simulink model "atrias_nmm_hardware"  (R2014b)
settings: Solver=ode4  StartTime=0.0  StopTime=inf  FixedStep=sample_time  RelTol=1e-3
undefined symbols (not defined in the file): A_lpf_dtau, B1_lpf_dtau, B2_lpf_dtau, boom_mount_angle, boom_pelvis_offset_angle, c, c_jointstop, contactThr, control_start_time, D12_T, d_y_boom_com_offset, d_y_boom_hip_offset, eref, fcut_contact, FmaxBFSH, FmaxGLU, FmaxHAM, FmaxHFL, FmaxRF, FmaxVAS, g, h_boom, HIP_MTR_MAX_CONT_TORQUE, initial_com_height, initial_dx, K, k_sea, kd_lateral, kd_phi12, kd_phi23, kp_lateral, kp_phi12, kp_phi23, l_boom_projected, L_distribution_switch, L_force_ctrl_switch, L_hip_trq_desired, L_knee_trq_desired, L_sea_input_switch, l_seg, L_stim_gain, L_stim_switch, l_yaw_center_to_pelvis, lambdaHip, lambdaKnee, lateral_offset, lateral_target_angle_left, lateral_target_angle_right, lateral_transition_force, loptBFSH, loptGLU, loptHAM, loptHFL, loptRF, loptVAS, Lphi12_des, Lphi23_des, lslackBFSH, lslackGLU, lslackHAM ... (+69)
libraries: simulink_extras x15, simulink x5, slrtlib x3
(part 9 of 9)

== matlab function atrias_nmm_hardware/Control/Behavior Control/Lateral Control ==
  data: tau_r output size=1; qLateralR input; dqLateralR input; qLateralL input; dqLateralL input; F_leg_R input; F_leg_L input; L_leg_R input; L_leg_L input; lateral_transition_force parameter; lateral_target_angle_right parameter; lateral_target_angle_left parameter; boom_mount_angle parameter; boom_pelvis_offset_angle parameter; l_yaw_center_to_pelvis parameter; m_leg_motor parameter; g parameter; lateral_offset parameter; tau_l output size=1; kp_lateral parameter; kd_lateral parameter; minimum_lateral_angle parameter; maximum_lateral_angle parameter; HIP_MTR_MAX_CONT_TORQUE parameter
function [tau_r, tau_l] = LateralBoomControl(qLateralR, dqLateralR, qLateralL, dqLateralL, F_leg_R, F_leg_L, L_leg_R, L_leg_L, lateral_transition_force, lateral_target_angle_right, lateral_target_angle_left, boom_mount_angle, boom_pelvis_offset_angle, l_yaw_center_to_pelvis, m_leg_motor, g, lateral_offset, kp_lateral, kd_lateral, minimum_lateral_angle, maximum_lateral_angle, HIP_MTR_MAX_CONT_TORQUE)

    gravity_compensation = m_leg_motor*g*lateral_offset;
    if (F_leg_R < lateral_transition_force && F_leg_L < lateral_transition_force), gravity_compensation = 0; end % freefall
    
    % Right Leg
    desired = saturate([lateral_target_angle_right, 0],minimum_lateral_angle,maximum_lateral_angle);
    measured = [qLateralR, dqLateralR];
    tau_r = [kp_lateral, kd_lateral] * (desired-measured)' + gravity_compensation;
    tau_r = max(min(HIP_MTR_MAX_CONT_TORQUE, tau_r),-HIP_MTR_MAX_CONT_TORQUE);
    
    if (F_leg_R >= lateral_transition_force)
        angle = qLateralR - boom_pelvis_offset_angle + boom_mount_angle;
        J =   (L_leg_R - l_yaw_center_to_pelvis*sin(angle)) ./ (L_leg_R.*l_yaw_center_to_pelvis.*cos(angle) - l_yaw_center_to_pelvis*lateral_offset*sin(angle));    
        tau_r = -F_leg_R*(J - lateral_offset) + gravity_compensation;
    end
    
    % Left Leg
    desired = saturate([lateral_target_angle_left, 0],minimum_lateral_angle,maximum_lateral_angle);
    measured = [qLateralL, dqLateralL];
    tau_l = [kp_lateral, kd_lateral] * (desired-measured)' + gravity_compensation;
    tau_l = max(min(HIP_MTR_MAX_CONT_TORQUE, tau_l),-HIP_MTR_MAX_CONT_TORQUE);
    
    if (F_leg_L >= lateral_transition_force)
        angle = qLateralL + boom_pelvis_offset_angle - boom_mount_angle;
        J =  -(L_leg_L + l_yaw_center_to_pelvis*sin(angle)) ./ (L_leg_L.*l_yaw_center_to_pelvis.*cos(angle) - l_yaw_center_to_pelvis*lateral_offset*sin(angle));  
        tau_l = F_leg_L*(J - lateral_offset) + gravity_compensation;  
    end
    
    % Stance
%     if ~escape
%         if ~placement && right_or_left
%             angle = qLateralR - boom_pelvis_offset_angle + boom_mount_angle;
%             J =   (l_leg - l_yaw_center_to_pelvis*sin(angle)) ./ (l_leg.*l_yaw_center_to_pelvis.*cos(angle) - l_yaw_center_to_pelvis*lateral_offset*sin(angle));    
%             tau_r = -F_leg*(J - lateral_offset) + gravity_compensation; % + lateral_offset ???  -F*(J+r) + g       F*(J-r) + g
%         elseif ~placement && ~right_or_left
%             angle = qLateralL + boom_pelvis_offset_angle - boom_mount_angle;
%             J =  -(l_leg + l_yaw_center_to_pelvis*sin(angle)) ./ (l_leg.*l_yaw_center_to_pelvis.*cos(angle) - l_yaw_center_to_pelvis*lateral_offset*sin(angle));  
%             tau_l = F_leg*(J - lateral_offset) + gravity_compensation;
%         end
%     end
end

function [desired_saturated] = saturate(desired, minimum_lateral_angle, maximum_lateral_angle)
    desired_saturated = desired;
    if desired(1) < minimum_lateral_angle
        desired_saturated = [minimum_lateral_angle, 0];
    elseif desired(1) > maximum_lateral_angle
        desired_saturated = [maximum_lateral_angle, 0];    
    end
end
